simulink model "Time_Gap"  (R2022b)
settings: configuration reference "CommonModelConfiguration" (kept outside this file)
undefined symbols (not defined in the file): cc_param_23, cc_param_311, cc_param_314, LCFG_DSF_Timeout2, LCFG_TG_Animation, LCFG_TG_MaxTG, LCFG_TG_MinTG
settings Model: Creator=rkallum  LastModifiedBy=OTHOMSO1
settings ConfigSetRef: SourceName=CommonModelConfiguration  SourceLocation=Base Workspace

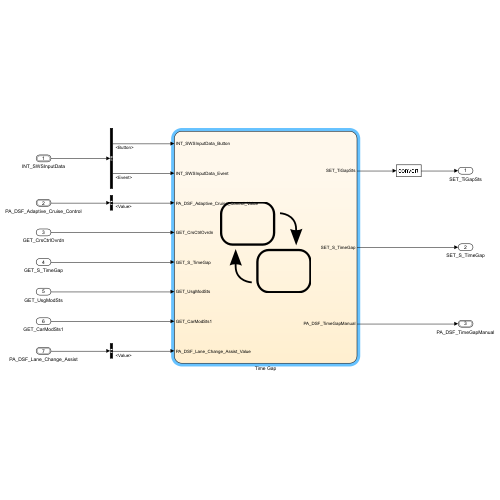
[thumbnail: Simulink's stored preview of the top-level diagram]
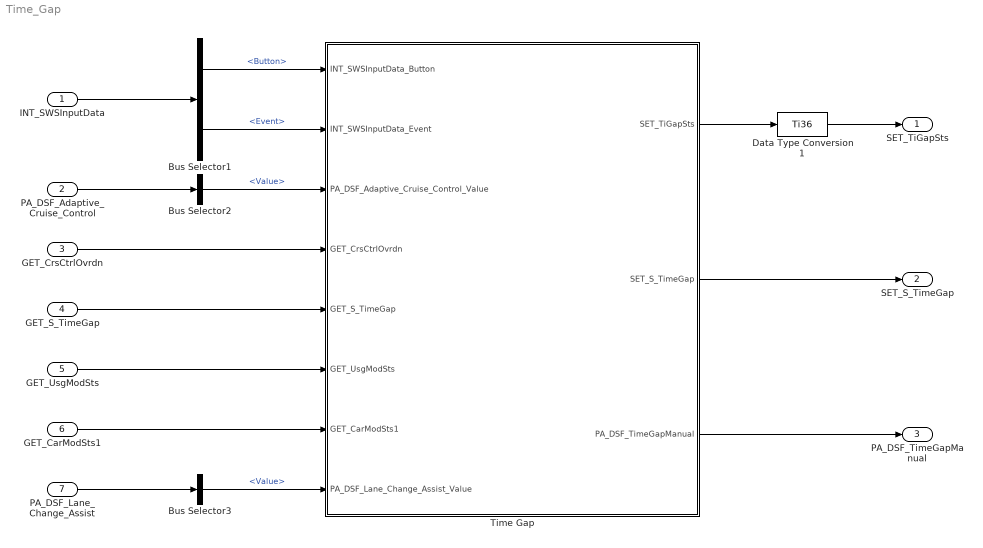
== system Time_Gap ==
  INT_SWSInputData : Inport  OutDataTypeStr=Bus: SWSInputData
  PA_DSF_Adaptive_Cruise_Control : Inport  Port=2  OutDataTypeStr=Bus: PA_DSF_ACC  SampleTime=1
  GET_CrsCtrlOvrdn : Inport  Port=3  OutDataTypeStr=Enum: OnOff1  SampleTime=1
  GET_S_TimeGap : Inport  Port=4  OutDataTypeStr=double  SampleTime=1
  GET_UsgModSts : Inport  Port=5  OutDataTypeStr=Enum: UsgModSts1  SampleTime=1
  GET_CarModSts1 : Inport  Port=6  OutDataTypeStr=Enum: CarModSts1
  PA_DSF_Lane_Change_Assist : Inport  Port=7  OutDataTypeStr=Bus: PA_DSF_LCA
  Bus Selector1 : BusSelector  OutputSignals=Button,Event
  Bus Selector2 : BusSelector  OutputSignals=Value
  Bus Selector3 : BusSelector  OutputSignals=Value
  Data Type Conversion1 : DataTypeConversion  OutDataTypeStr=Ti36  SaturateOnIntegerOverflow=off  RndMeth=Floor
  Time Gap : Stateflow chart  TreatAsAtomicUnit=on
  SET_TiGapSts : Outport  OutDataTypeStr=Ti36  VectorParamsAs1DForOutWhenUnconnected=off
  SET_S_TimeGap : Outport  Port=2  OutDataTypeStr=double  VectorParamsAs1DForOutWhenUnconnected=off
  PA_DSF_TimeGapManual : Outport  Port=3  OutDataTypeStr=Bus: PA_DSF_TimeGapManual  VectorParamsAs1DForOutWhenUnconnected=off
  wires:
  GET_UsgModSts/1 -> Time Gap/6(GET_UsgModSts)
  GET_CarModSts1/1 -> Time Gap/7(GET_CarModSts1)
  Bus Selector1/1 -> Time Gap/1(INT_SWSInputData_Button)  "<Button>"
  Bus Selector1/2 -> Time Gap/2(INT_SWSInputData_Event)  "<Event>"
  INT_SWSInputData/1 -> Bus Selector1/1
  Bus Selector2/1 -> Time Gap/3(PA_DSF_Adaptive_Cruise_Control_Value)  "<Value>"
  PA_DSF_Adaptive_Cruise_Control/1 -> Bus Selector2/1
  GET_CrsCtrlOvrdn/1 -> Time Gap/4(GET_CrsCtrlOvrdn)
  GET_S_TimeGap/1 -> Time Gap/5(GET_S_TimeGap)
  Time Gap/1(SET_TiGapSts) -> Data Type Conversion1/1
  Data Type Conversion1/1 -> SET_TiGapSts/1
  Time Gap/2(SET_S_TimeGap) -> SET_S_TimeGap/1
  Time Gap/3(PA_DSF_TimeGapManual) -> PA_DSF_TimeGapManual/1
  PA_DSF_Lane_Change_Assist/1 -> Bus Selector3/1
  Bus Selector3/1 -> Time Gap/8(PA_DSF_Lane_Change_Assist_Value)  "<Value>"

== stateflow chart Time_Gap/Time Gap ==
  state CARCONFIG_INVALID
    entry:
    SET_TiGapSts = GET_S_TimeGap;
    SET_S_TimeGap = SET_TiGapSts;
    PA_DSF_TimeGapManual.Status = E_CommonStatus.NotPresent;
    PA_DSF_TimeGapManual.Value = E_DSF_TG(GET_S_TimeGap);
    PA_DSF_TimeGapManual.Action = E_DSF_TG_Action.No_Action;
  state SYSTEM_OK
    state isActive = ActivationCheck [function]
      (default) -> (junction 54)
      (junction 54) -> (junction 55) [order 1] : [GET_CarModSts1==CarModSts1.CarModSts1_CarModNorm &&...
          | GET_UsgModSts==UsgModSts1.UsgModSts1_UsgModDrvg]
      (junction 54) -> (junction 56) [order 2] : {isActive=false;}
      (junction 55) -> (junction 57) : {isActive=true;}
      (junction 57) -> (junction 56)
      (junction 56) -> (junction 58)
    state NOT_ACTIVE
      entry:
      SET_TiGapSts = GET_S_TimeGap;
      SET_S_TimeGap = SET_TiGapSts;
      PA_DSF_TimeGapManual.Value = E_DSF_TG(GET_S_TimeGap);
      PA_DSF_TimeGapManual.Action = E_DSF_TG_Action.No_Action;
      PA_DSF_TimeGapManual.Status = E_CommonStatus.Disabled;
    state ACTIVE
      entry:
      SET_TiGapSts = GET_S_TimeGap;
      SET_S_TimeGap = SET_TiGapSts;
      PA_DSF_TimeGapManual.Value = E_DSF_TG(GET_S_TimeGap);
      PA_DSF_TimeGapManual.Action = E_DSF_TG_Action.No_Action;
      state MIN_MAX_TG [parallel]
        settings: executionOrder=1
        (default) -> (junction 722)
        (junction 722) -> (junction 723) [order 1] : %Argus3
            | [cc_param_311==3]
        (junction 722) -> (junction 778) [order 2] : {MinTG = 1;
            | MaxTG = 5;}
        (junction 723) -> (junction 777) : {MinTG = 1;
            | MaxTG = 3;}
        (junction 777) -> (junction 778)
        (junction 778) -> (junction 779)
      state BUS_SIGNALS [parallel]
        entry:
        animateTG = false;
        settings: executionOrder=2
        state retval = PreCondition [function]
          (default) -> (junction 458)
          (junction 458) -> (junction 459) [order 1] : [(PA_DSF_Adaptive_Cruise_Control_Value==E_DSF_Value.DSF_Active &&...
              | GET_CrsCtrlOvrdn==OnOff1.OnOff1_Off)]
          (junction 458) -> (junction 460) [order 2] : {retval=false}
          (junction 459) -> (junction 461) : {retval=true}
          (junction 461) -> (junction 460)
          (junction 460) -> (junction 462)
        state IGNORE_INPUT
        state APPLY_INPUT
          APPLY_INPUT -> (junction 628) [order 1]
          (junction 628) -> (junction 629) [order 1] : [hasChanged(GET_S_TimeGap) &&...
              | SET_TiGapSts~=GET_S_TimeGap]
          (junction 628) -> (junction 630) [order 2]
          (junction 629) -> (junction 631) : {SET_TiGapSts = GET_S_TimeGap;
              | SET_S_TimeGap = SET_TiGapSts;
              | showTG = true;}
          (junction 631) -> (junction 630)
          (junction 630) -> (junction 632)
          (junction 632) -> (junction 633) [order 1] : [hasChangedTo(INT_SWSInputData_Event,E_SWSEvent.Push) &&...
              | (INT_SWSInputData_Button==E_SWSButton.BtnL6Req ||...
              | INT_SWSInputData_Button==E_SWSButton.BtnL7Req)]
              | {showTG = true;}
          (junction 633) -> (junction 635)
          (junction 632) -> (junction 637) [order 2]
          (junction 635) -> (junction 634) [order 2] : [INT_SWSInputData_Button==...
              | E_SWSButton.BtnL6Req &&...
              | SET_TiGapSts>MinTG]
          (junction 635) -> (junction 636) [order 1] : [INT_SWSInputData_Button==...
              | E_SWSButton.BtnL7Req &&...
              | SET_TiGapSts<MaxTG]
          (junction 634) -> (junction 638) : {SET_TiGapSts = SET_TiGapSts - 1;
              | SET_S_TimeGap = SET_TiGapSts;}
          (junction 635) -> (junction 639) [order 3] : {animateTG = true;}
          (junction 636) -> (junction 640) : {SET_TiGapSts = SET_TiGapSts + 1;
              | SET_S_TimeGap = SET_TiGapSts;}
          (junction 638) -> (junction 637)
          (junction 639) -> (junction 638)
          (junction 640) -> (junction 639)
          (junction 637) -> (junction 641)
        (default) -> (junction 660)
        (junction 660) -> (junction 620) [order 1] : [PreCondition]
        (junction 660) -> IGNORE_INPUT [order 2]
        (junction 620) -> APPLY_INPUT
        IGNORE_INPUT -> APPLY_INPUT : [PreCondition]
        APPLY_INPUT -> IGNORE_INPUT [order 1] : [~PreCondition]
      state PUBLIC_ATTRIBUTE [parallel]
        settings: executionOrder=3
        state ACC_OFF
          entry:
          PA_DSF_TimeGapManual.Action = E_DSF_TG_Action.No_Action;
          entry, during:
          setStopModeMan();
          state setStopModeMan [function]
            (default) -> (junction 544)
            (junction 544) -> (junction 543) [order 1] : %Show TG during stop mode for pre-Argus3
                | [PA_DSF_Adaptive_Cruise_Control_Value==E_DSF_Value.DSF_StopMode &&...
                | cc_param_311~=3]
            (junction 544) -> (junction 546) [order 2] : {PA_DSF_TimeGapManual.Status = E_CommonStatus.Disabled;}
            (junction 543) -> (junction 545) : {PA_DSF_TimeGapManual.Status = E_CommonStatus.Available;}
            (junction 545) -> (junction 546)
            (junction 546) -> (junction 547)
        state ACC
          entry:
          PA_DSF_TimeGapManual.Status = E_CommonStatus.Available;
          showTG = true;
          state ACTION [parallel]
            settings: executionOrder=1
            state DECREASE
              entry:
              PA_DSF_TimeGapManual.Action = E_DSF_TG_Action.Decrease;
            state NO_ACTION
              entry:
              PA_DSF_TimeGapManual.Action = E_DSF_TG_Action.No_Action;
            state INCREASE
              entry:
              PA_DSF_TimeGapManual.Action = E_DSF_TG_Action.Increase;
            NO_ACTION -> DECREASE [order 1] : [animateTG &&...
                | SET_TiGapSts==E_DSF_TG(MinTG) &&...
                | GET_CrsCtrlOvrdn==OnOff1.OnOff1_Off]
            DECREASE -> NO_ACTION : [after(LCFG_TG_Animation,sec)]
            (default) -> NO_ACTION
            INCREASE -> NO_ACTION : [after(LCFG_TG_Animation,sec)]
            NO_ACTION -> INCREASE [order 2] : [animateTG &&...
                | SET_TiGapSts==E_DSF_TG(MaxTG) &&...
                | GET_CrsCtrlOvrdn==OnOff1.OnOff1_Off]
          state VALUE [parallel]
            settings: executionOrder=2
            state activeLCA = isActiveLCA [function]
              (default) -> (junction 680)
              (junction 680) -> (junction 681) [order 1] : [PA_DSF_Lane_Change_Assist_Value==E_DSF_LCA.LCA_Executing ||...
                  | PA_DSF_Lane_Change_Assist_Value==E_DSF_LCA.LCA_Aborted ||...
                  | PA_DSF_Lane_Change_Assist_Value==E_DSF_LCA.LCA_Cancelled]
              (junction 680) -> (junction 682) [order 2] : {activeLCA = false;}
              (junction 681) -> (junction 683) : {activeLCA = true;}
              (junction 683) -> (junction 682)
              (junction 682) -> (junction 684)
            state HIDE_TG
              entry:
              PA_DSF_TimeGapManual.Value =...
              E_DSF_TG.TimeGap_0;
            state SHOW_TG
              (default) -> (junction 693)
              (junction 693) -> (junction 694) [order 1] : [SET_TiGapSts==1]
                  | {PA_DSF_TimeGapManual.Value = E_DSF_TG.TimeGap_1;}
              (junction 693) -> (junction 695) [order 2]
              (junction 694) -> (junction 696)
              (junction 695) -> (junction 696) [order 1] : [SET_TiGapSts==2]
                  | {PA_DSF_TimeGapManual.Value = E_DSF_TG.TimeGap_2;}
              (junction 695) -> (junction 697) [order 2]
              (junction 696) -> (junction 698)
              (junction 697) -> (junction 698) [order 1] : [SET_TiGapSts==3]
                  | {PA_DSF_TimeGapManual.Value = E_DSF_TG.TimeGap_3;}
              (junction 697) -> (junction 699) [order 2]
              (junction 698) -> (junction 700)
              (junction 699) -> (junction 700) [order 1] : [SET_TiGapSts==4]
                  | {PA_DSF_TimeGapManual.Value = E_DSF_TG.TimeGap_4;}
              (junction 699) -> (junction 701) [order 2] : {PA_DSF_TimeGapManual.Value = E_DSF_TG.TimeGap_5;}
              (junction 700) -> (junction 702)
              (junction 702) -> (junction 701)
              (junction 701) -> (junction 703)
            (default) -> (junction 672)
            (junction 672) -> HIDE_TG [order 2]
            (junction 672) -> SHOW_TG [order 1] : %Show time gap always if not Argus3
                | [(showTG && ~isActiveLCA) || cc_param_311~=3]
            HIDE_TG -> SHOW_TG : [showTG && ~isActiveLCA ||...
                | cc_param_311~=3]
            SHOW_TG -> HIDE_TG : %Show time gap always if not Argus3
                | [(after(LCFG_DSF_Timeout2, sec) ||...
                | isActiveLCA) && cc_param_311==3]
                | {showTG = false;}
        (default) -> (junction 409)
        (junction 409) -> (junction 412) [order 1] : [PA_DSF_Adaptive_Cruise_Control_Value~=E_DSF_Value.DSF_Active]
        (junction 409) -> ACC [order 2]
        (junction 412) -> ACC_OFF
        ACC -> ACC_OFF : [PA_DSF_Adaptive_Cruise_Control_Value~=E_DSF_Value.DSF_Active]
        ACC_OFF -> ACC : [PA_DSF_Adaptive_Cruise_Control_Value==E_DSF_Value.DSF_Active]
    (default) -> (junction 443)
    (junction 443) -> NOT_ACTIVE [order 1] : [~ActivationCheck()]
    (junction 443) -> (junction 446) [order 2]
    NOT_ACTIVE -> ACTIVE : [ActivationCheck()]
    ACTIVE -> NOT_ACTIVE : [~ActivationCheck()]
    (junction 446) -> ACTIVE
  (default) -> (junction 4)
  (junction 4) -> CARCONFIG_INVALID [order 2]
  (junction 4) -> SYSTEM_OK [order 1] : [cc_param_23>2]
  data: isActive function_output boolean; retval function_output; activeLCA function_output; cc_param_23 parameter; INT_SWSInputData_Button input Enum: E_SWSButton; INT_SWSInputData_Event input Enum: E_SWSEvent; PA_DSF_Adaptive_Cruise_Control_Value input Enum: E_DSF_Value; GET_CrsCtrlOvrdn input Enum: OnOff1; SET_TiGapSts output double; GET_S_TimeGap input double; SET_S_TimeGap output double; GET_UsgModSts input Enum: UsgModSts1; GET_CarModSts1 input Enum: CarModSts1; LCFG_TG_MaxTG parameter; LCFG_TG_MinTG parameter; cc_param_314 parameter; PA_DSF_TimeGapManual output Bus: PA_DSF_TimeGapManual =0; LCFG_TG_Animation parameter; showTG local boolean; PA_DSF_Lane_Change_Assist_Value input; LCFG_DSF_Timeout2 parameter; cc_param_311 parameter; MinTG local; MaxTG local; animateTG local
